simulink model "BypassSerialBlockTest"  (R2025b)
settings: Solver=FixedStepAuto  StartTime=0.0  StopTime=inf  FixedStep=.01  RelTol=1e-3
libraries: simulink x2
settings Model: Creator=talles  LastModifiedBy=ajax

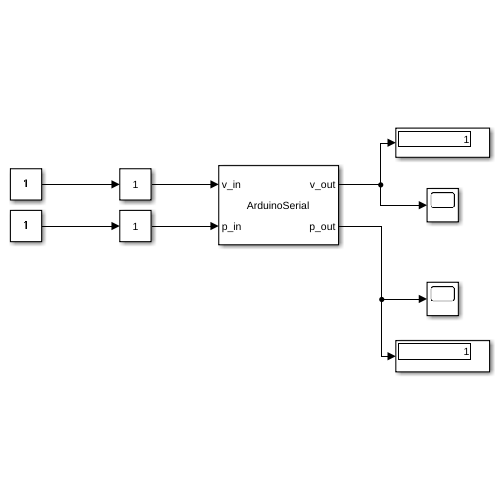
[thumbnail: Simulink's stored preview of the top-level diagram]
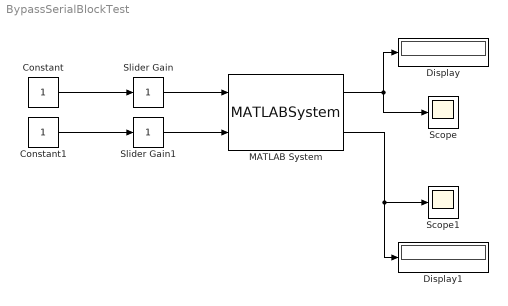
== system BypassSerialBlockTest ==
  Constant : Constant
  Constant1 : Constant
  Display : Display
  Display1 : Display
  MATLAB System : MATLABSystem  System=ArduinoSerial  COMPort=/dev/ttyACM0  BaudRate=115200  SimulateUsing=Interpreted execution
      mask Type: ArduinoSerial
  Scope : Scope
      settings: ActiveDisplayYMinimum=-1  ActiveDisplayYMaximum=1
  Scope1 : Scope
      settings: ActiveDisplayYMinimum=-0.24999999999999994  ActiveDisplayYMaximum=2.25
  Slider Gain : simulink/Math Operations/Slider Gain  gain=1  low=0  high=2
  Slider Gain1 : simulink/Math Operations/Slider Gain  gain=1  low=0  high=2
  wires:
  MATLAB System/1 -> Scope/1, Display/1
  MATLAB System/2 -> Display1/1, Scope1/1
  Slider Gain1/1 -> MATLAB System/2
  Constant1/1 -> Slider Gain1/1
  Constant/1 -> Slider Gain/1
  Slider Gain/1 -> MATLAB System/1
